simulink model "uloha_simulink"  (R2017b)
settings: Solver=VariableStepAuto  StartTime=0.0  StopTime=60  RelTol=1e-3
settings Model: Creator=jan.sedivy  LastModifiedBy=jan.sedivy

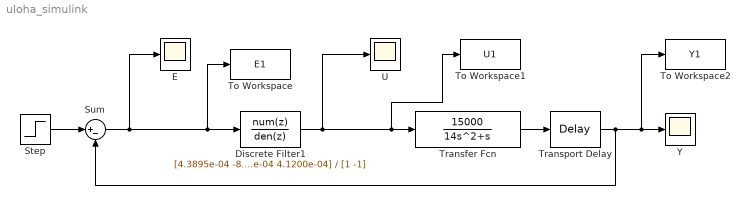
== system uloha_simulink ==
  Discrete Filter1 : DiscreteFilter  Numerator=[4.3895e-04 -8.5095e-04 4.1200e-04]  Denominator=[1 -1]  SampleTime=1
  "E " : Scope
  Step : Step  Time=0  SampleTime=0
  Sum : Sum  Inputs=|+-
  To Workspace : ToWorkspace  VariableName=E1  SaveFormat=Timeseries  SampleTime=-1
  To Workspace1 : ToWorkspace  VariableName=U1  SaveFormat=Timeseries  SampleTime=-1
  To Workspace2 : ToWorkspace  VariableName=Y1  SaveFormat=Timeseries  SampleTime=-1
  Transfer Fcn : TransferFcn  Numerator=[15000]  Denominator=[14 1 0]
  Transport Delay : TransportDelay
  "U " : Scope
  "Y " : Scope
  wires:
  Discrete Filter1/1 -> "U "/1, To Workspace1/1, Transfer Fcn/1
  Transport Delay/1 -> Sum/2, To Workspace2/1, "Y "/1
  Sum/1 -> Discrete Filter1/1, To Workspace/1, "E "/1
  Transfer Fcn/1 -> Transport Delay/1
  Step/1 -> Sum/1
